simulink model "PID_controllers_without_disturbance"  (R2018a)
settings: Solver=VariableStepAuto  StartTime=0.0  StopTime=80  RelTol=1e-3
libraries: simulink x4
settings Model: Creator=Wa'el WMJ  LastModifiedBy=Wa'el WMJ
settings DataIOCC: ReturnWorkspaceOutputs=on
settings DebuggingCC: UnconnectedInputMsg=none  UnconnectedOutputMsg=none  UnconnectedLineMsg=none
settings ModelReferenceCC: EnableRefExpFcnMdlSchedulingChecks=off
settings SFSimCC: SimUseLocalCustomCode=on
settings RTWCC: Description=Generic Real-Time Target  RTWUseLocalCustomCode=on

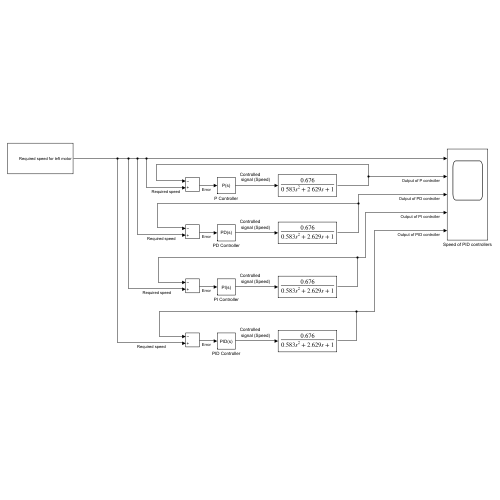
[thumbnail: Simulink's stored preview of the top-level diagram]
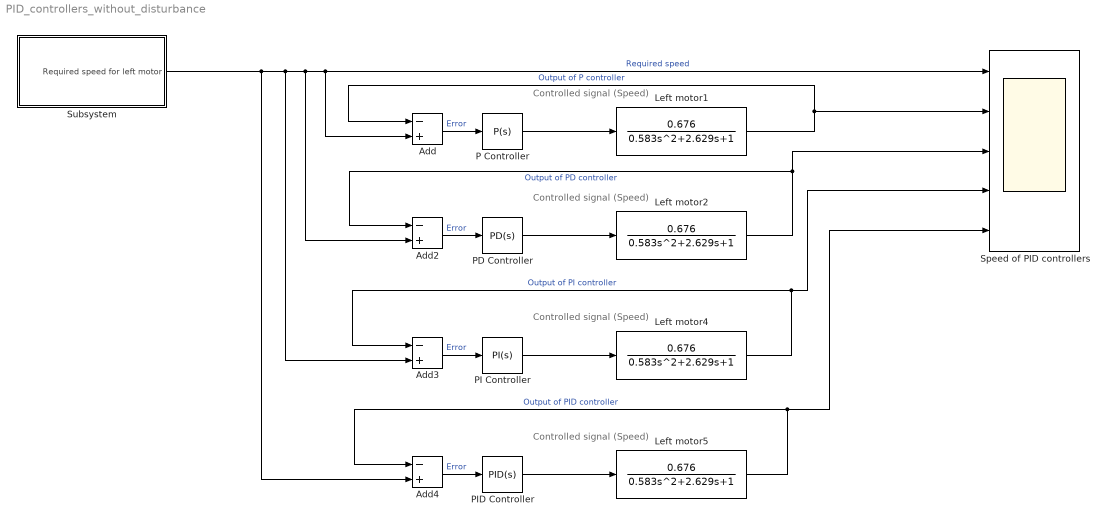
== system PID_controllers_without_disturbance ==
  note: Controlled
      | signal (Speed)
  note: Controlled
      | signal (Speed)
  note: Controlled
      | signal (Speed)
  note: Controlled
      | signal (Speed)
  Add{,2..4} (4 alike) : Sum  Inputs=-+
  Left motor{1..2,4..5} (4 alike) : TransferFcn  Numerator=[0.676]  Denominator=[0.583 2.629 1]
  P Controller : simulink/Continuous/PID Controller  Controller=P  Form=Parallel  TimeDomain=Continuous-time  SampleTime=-1  IntegratorMethod=Forward Euler  ControllerParametersSource=internal  P=2.52450586857171  I=1.66493394941622  D=0.2823545342518  N=86.8800086214376  UseFilter=on  TunerSelectOption=Transfer Function Based (PID Tuner App)  InitialConditionSource=internal  InitialConditionForIntegrator=0  InitialConditionForFilter=0  DifferentiatorICPrevScaledInput=0  ExternalReset=none  TrackingMode=off  Kt=1  LimitOutput=off  UpperSaturationLimit=inf  LowerSaturationLimit=-inf  LinearizeAsGain=on  AntiWindupMode=none  Kb=1  POutMin=[]  POutMax=[]  IOutMin=[]  IOutMax=[]  DOutMin=[]  DOutMax=[]  NOutMin=[]  NOutMax=[]  SumOutMin=[]  SumOutMax=[]  SaturationOutMin=[]  SaturationOutMax=[]  PParamMin=[]  PParamMax=[]  IParamMin=[]  IParamMax=[]  DParamMin=[]  DParamMax=[]  NParamMin=[]  NParamMax=[]  KbParamMin=[]  KbParamMax=[]  KtParamMin=[]  KtParamMax=[]  KbOutMin=[]  KbOutMax=[]  KtOutMin=[]  KtOutMax=[]  IntegratorOutMin=[]  IntegratorOutMax=[]  FilterOutMin=[]  FilterOutMax=[]  SumI1OutMin=[]  SumI1OutMax=[]  SumI2OutMin=[]  SumI2OutMax=[]  SumI3OutMin=[]  SumI3OutMax=[]  SumDOutMin=[]  SumDOutMax=[]  DifferentiatorOutMin=[]  DifferentiatorOutMax=[]  FilterDiffOutCoefMin=[]  FilterDiffOutCoefMax=[]  ReciprocalOutMin=[]  ReciprocalOutMax=[]  SumDenOutMin=[]  SumDenOutMax=[]  SumNumOutMin=[]  SumNumOutMax=[]  DivideOutMin=[]  DivideOutMax=[]  IntegratorContinuousStateAttributes=''  IntegratorStateMustResolveToSignalObject=off  IntegratorRTWStateStorageClass=Auto  FilterContinuousStateAttributes=''  FilterStateMustResolveToSignalObject=off  FilterRTWStateStorageClass=Auto
  PD Controller : simulink/Continuous/PID Controller  Controller=PD  Form=Parallel  TimeDomain=Continuous-time  SampleTime=-1  IntegratorMethod=Forward Euler  ControllerParametersSource=internal  P=2.41347213312579  I=1.66493394941622  D=0  N=100  UseFilter=on  TunerSelectOption=Transfer Function Based (PID Tuner App)  InitialConditionSource=internal  InitialConditionForIntegrator=0  InitialConditionForFilter=0  DifferentiatorICPrevScaledInput=0  ExternalReset=none  TrackingMode=off  Kt=1  LimitOutput=off  UpperSaturationLimit=inf  LowerSaturationLimit=-inf  LinearizeAsGain=on  AntiWindupMode=none  Kb=1  POutMin=[]  POutMax=[]  IOutMin=[]  IOutMax=[]  DOutMin=[]  DOutMax=[]  NOutMin=[]  NOutMax=[]  SumOutMin=[]  SumOutMax=[]  SaturationOutMin=[]  SaturationOutMax=[]  PParamMin=[]  PParamMax=[]  IParamMin=[]  IParamMax=[]  DParamMin=[]  DParamMax=[]  NParamMin=[]  NParamMax=[]  KbParamMin=[]  KbParamMax=[]  KtParamMin=[]  KtParamMax=[]  KbOutMin=[]  KbOutMax=[]  KtOutMin=[]  KtOutMax=[]  IntegratorOutMin=[]  IntegratorOutMax=[]  FilterOutMin=[]  FilterOutMax=[]  SumI1OutMin=[]  SumI1OutMax=[]  SumI2OutMin=[]  SumI2OutMax=[]  SumI3OutMin=[]  SumI3OutMax=[]  SumDOutMin=[]  SumDOutMax=[]  DifferentiatorOutMin=[]  DifferentiatorOutMax=[]  FilterDiffOutCoefMin=[]  FilterDiffOutCoefMax=[]  ReciprocalOutMin=[]  ReciprocalOutMax=[]  SumDenOutMin=[]  SumDenOutMax=[]  SumNumOutMin=[]  SumNumOutMax=[]  DivideOutMin=[]  DivideOutMax=[]  IntegratorContinuousStateAttributes=''  IntegratorStateMustResolveToSignalObject=off  IntegratorRTWStateStorageClass=Auto  FilterContinuousStateAttributes=''  FilterStateMustResolveToSignalObject=off  FilterRTWStateStorageClass=Auto
  PI Controller : simulink/Continuous/PID Controller  Controller=PI  Form=Parallel  TimeDomain=Continuous-time  SampleTime=-1  IntegratorMethod=Forward Euler  ControllerParametersSource=internal  P=2.31547573896949  I=1.63494454176496  D=0  N=100  UseFilter=on  TunerSelectOption=Transfer Function Based (PID Tuner App)  InitialConditionSource=internal  InitialConditionForIntegrator=0  InitialConditionForFilter=0  DifferentiatorICPrevScaledInput=0  ExternalReset=none  TrackingMode=off  Kt=1  LimitOutput=off  UpperSaturationLimit=inf  LowerSaturationLimit=-inf  LinearizeAsGain=on  AntiWindupMode=none  Kb=1  POutMin=[]  POutMax=[]  IOutMin=[]  IOutMax=[]  DOutMin=[]  DOutMax=[]  NOutMin=[]  NOutMax=[]  SumOutMin=[]  SumOutMax=[]  SaturationOutMin=[]  SaturationOutMax=[]  PParamMin=[]  PParamMax=[]  IParamMin=[]  IParamMax=[]  DParamMin=[]  DParamMax=[]  NParamMin=[]  NParamMax=[]  KbParamMin=[]  KbParamMax=[]  KtParamMin=[]  KtParamMax=[]  KbOutMin=[]  KbOutMax=[]  KtOutMin=[]  KtOutMax=[]  IntegratorOutMin=[]  IntegratorOutMax=[]  FilterOutMin=[]  FilterOutMax=[]  SumI1OutMin=[]  SumI1OutMax=[]  SumI2OutMin=[]  SumI2OutMax=[]  SumI3OutMin=[]  SumI3OutMax=[]  SumDOutMin=[]  SumDOutMax=[]  DifferentiatorOutMin=[]  DifferentiatorOutMax=[]  FilterDiffOutCoefMin=[]  FilterDiffOutCoefMax=[]  ReciprocalOutMin=[]  ReciprocalOutMax=[]  SumDenOutMin=[]  SumDenOutMax=[]  SumNumOutMin=[]  SumNumOutMax=[]  DivideOutMin=[]  DivideOutMax=[]  IntegratorContinuousStateAttributes=''  IntegratorStateMustResolveToSignalObject=off  IntegratorRTWStateStorageClass=Auto  FilterContinuousStateAttributes=''  FilterStateMustResolveToSignalObject=off  FilterRTWStateStorageClass=Auto
  PID Controller : simulink/Continuous/PID Controller  Controller=PID  Form=Parallel  TimeDomain=Continuous-time  SampleTime=-1  IntegratorMethod=Forward Euler  ControllerParametersSource=internal  P=2.40661634890179  I=1.66493394941622  D=0.2823545342518  N=86.8800086214376  UseFilter=on  TunerSelectOption=Transfer Function Based (PID Tuner App)  InitialConditionSource=internal  InitialConditionForIntegrator=0  InitialConditionForFilter=0  DifferentiatorICPrevScaledInput=0  ExternalReset=none  TrackingMode=off  Kt=1  LimitOutput=off  UpperSaturationLimit=inf  LowerSaturationLimit=-inf  LinearizeAsGain=on  AntiWindupMode=none  Kb=1  POutMin=[]  POutMax=[]  IOutMin=[]  IOutMax=[]  DOutMin=[]  DOutMax=[]  NOutMin=[]  NOutMax=[]  SumOutMin=[]  SumOutMax=[]  SaturationOutMin=[]  SaturationOutMax=[]  PParamMin=[]  PParamMax=[]  IParamMin=[]  IParamMax=[]  DParamMin=[]  DParamMax=[]  NParamMin=[]  NParamMax=[]  KbParamMin=[]  KbParamMax=[]  KtParamMin=[]  KtParamMax=[]  KbOutMin=[]  KbOutMax=[]  KtOutMin=[]  KtOutMax=[]  IntegratorOutMin=[]  IntegratorOutMax=[]  FilterOutMin=[]  FilterOutMax=[]  SumI1OutMin=[]  SumI1OutMax=[]  SumI2OutMin=[]  SumI2OutMax=[]  SumI3OutMin=[]  SumI3OutMax=[]  SumDOutMin=[]  SumDOutMax=[]  DifferentiatorOutMin=[]  DifferentiatorOutMax=[]  FilterDiffOutCoefMin=[]  FilterDiffOutCoefMax=[]  ReciprocalOutMin=[]  ReciprocalOutMax=[]  SumDenOutMin=[]  SumDenOutMax=[]  SumNumOutMin=[]  SumNumOutMax=[]  DivideOutMin=[]  DivideOutMax=[]  IntegratorContinuousStateAttributes=''  IntegratorStateMustResolveToSignalObject=off  IntegratorRTWStateStorageClass=Auto  FilterContinuousStateAttributes=''  FilterStateMustResolveToSignalObject=off  FilterRTWStateStorageClass=Auto
  Speed of PID controllers : Scope  NumInputPorts=5
  Subsystem : Subsystem
  wires:
  Left motor1/1 -> Speed of PID controllers/2, Add/1  "Output of P controller"
  Add/1 -> P Controller/1  "Error"
  P Controller/1 -> Left motor1/1
  PD Controller/1 -> Left motor2/1
  Left motor2/1 -> Add2/1, Speed of PID controllers/3  "Output of PD controller"
  Add2/1 -> PD Controller/1  "Error"
  Add3/1 -> PI Controller/1  "Error"
  PI Controller/1 -> Left motor4/1
  Left motor4/1 -> Speed of PID controllers/4, Add3/1  "Output of PI controller"
  PID Controller/1 -> Left motor5/1
  Left motor5/1 -> Speed of PID controllers/5, Add4/1  "Output of PID controller"
  Add4/1 -> PID Controller/1  "Error"
  Subsystem/1(Required speed for left motor) -> Add4/2, Add3/2, Add2/2, Speed of PID controllers/1, Add/2  "Required speed"

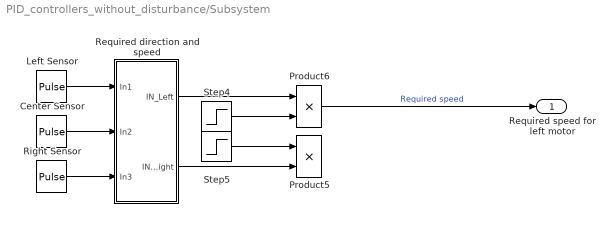
== system PID_controllers_without_disturbance/Subsystem ==
  "Center Sensor " : DiscretePulseGenerator  PulseType=Time based  Period=40  PulseWidth=50  PhaseDelay=20
  Left Sensor : DiscretePulseGenerator  PulseType=Time based  Period=80  PulseWidth=50  PhaseDelay=40
  Product5 : Product
  Product6 : Product
  Required direction and speed : Subsystem
  "Right Sensor " : DiscretePulseGenerator  PulseType=Time based  Period=20  PulseWidth=50  PhaseDelay=10
  Step4 : Step  Time=0  SampleTime=0
  Step5 : Step  Time=0  SampleTime=0
  Required speed for left motor : Outport
  wires:
  "Center Sensor "/1 -> Required direction and speed/2(In2)
  Left Sensor/1 -> Required direction and speed/1(In1)
  Product6/1 -> Required speed for left motor/1  "Required speed"
  Required direction and speed/2(IN_Right) -> Product5/2
  Step4/1 -> Product6/2
  Step5/1 -> Product5/1
  "Right Sensor "/1 -> Required direction and speed/3(In3)
  Required direction and speed/1(IN_Left) -> Product6/1

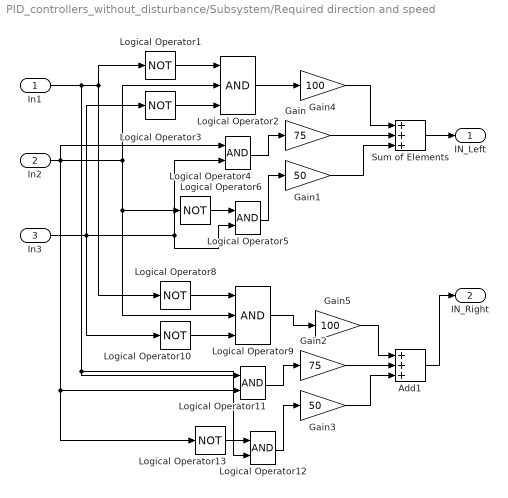
== system PID_controllers_without_disturbance/Subsystem/Required direction and speed ==
  In1 : Inport
  In2 : Inport  Port=2
  In3 : Inport  Port=3
  Add1 : Sum  Inputs=+++
  Gain : Gain  Gain=75
  Gain1 : Gain  Gain=50
  Gain2 : Gain  Gain=75
  Gain3 : Gain  Gain=50
  Gain4 : Gain  Gain=100
  Gain5 : Gain  Gain=100
  Logical Operator{1,3,6,8,10,13} (6 alike) : Logic  Operator=NOT  Inputs=3  AllPortsSameDT=off  OutDataTypeStr=boolean
  Logical Operator{4..5,11..12} (4 alike) : Logic  AllPortsSameDT=off  OutDataTypeStr=boolean
  Logical Operator2 : Logic  Inputs=3  AllPortsSameDT=off  OutDataTypeStr=boolean
  Logical Operator9 : Logic  Inputs=3  AllPortsSameDT=off  OutDataTypeStr=boolean
  Sum of Elements : Sum  Inputs=+++
  IN_Left : Outport
  IN_Right : Outport  Port=2
  wires:
  Logical Operator1/1 -> Logical Operator2/1
  Logical Operator3/1 -> Logical Operator2/3
  In1/1 -> Logical Operator12/2, Logical Operator11/1, Logical Operator8/1, Logical Operator1/1
  In2/1 -> Logical Operator13/1, Logical Operator11/2, Logical Operator4/1, Logical Operator9/2, Logical Operator6/1, Logical Operator2/2
  In3/1 -> Logical Operator10/1, Logical Operator5/2, Logical Operator4/2, Logical Operator3/1
  Logical Operator6/1 -> Logical Operator5/1
  Logical Operator4/1 -> Gain/1
  Logical Operator5/1 -> Gain1/1
  Logical Operator11/1 -> Gain2/1
  Gain2/1 -> Add1/2
  Logical Operator10/1 -> Logical Operator9/3
  Logical Operator8/1 -> Logical Operator9/1
  Gain3/1 -> Add1/3
  Logical Operator12/1 -> Gain3/1
  Logical Operator13/1 -> Logical Operator12/1
  Add1/1 -> IN_Right/1
  Sum of Elements/1 -> IN_Left/1
  Gain/1 -> Sum of Elements/2
  Gain1/1 -> Sum of Elements/3
  Gain4/1 -> Sum of Elements/1
  Logical Operator2/1 -> Gain4/1
  Gain5/1 -> Add1/1
  Logical Operator9/1 -> Gain5/1
